simulink model "rectifire_single_inverter_pv1"  (R2022b)
settings: Solver=ode23tb  StartTime=0  StopTime=3  RelTol=1e-4
undefined symbols (not defined in the file): Ion, Lithium, P_100, sigbuilder_block, time_step
libraries: spsSeriesRLCBranchLib x26, spsTriangleGeneratorLib x26, slpidlib x26, spsVoltageMeasurementLib x14, spsCurrentMeasurementLib x11, spsDiodeLib x9, simulink x8, spsIGBTDiodeLib x8, spsMosfetLib x8, powerlib_extras x4, spsGroundLib x2, spsBatteryLib x2
(part 6 of 6)

== matlab function rectifire_single_inverter_pv1/battery/Battery and DC-DC converter/MATLAB Function7 ==
  settings: updateMethod=DISCRETE
  data: iL_ref input; u1 output; iL input; vc_ref input; vc input; vin input; i_out input; Ts input; u2 output; Bus_load input
function [u1, u2] = Passivity_BC(iL_ref, iL, vc_ref, vc, vin, i_out, Ts, Bus_load)
% Constant output voltage Module
%   param vc_ref: expected
%   param vc: dcdc output voltage
%   param vin: input voltage
%   param io: current in output side
%   param Bus_load:
%% system parameters
L = 40e-6;  % Inductance 电感 20uH
L_DMinductor = 2.2e-6;
L = L + L_DMinductor;
RL = 0.004;
Co = 1440e-6;  % 电容大小

zeta1 = L / RL * 2000;  % dumping gains
zeta2 = Co * 1000; 

% if Bus_load > 1e4
%     zeta2 = 1e-3;
% end


% error functions: state variable
x1 = iL - iL_ref;
x2 = vc - vc_ref;
persistent iL_ref_old vc_ref_old;
if isempty(iL_ref_old)
    iL_ref_old = 0;
    vc_ref_old = 0;
end

diL_ref = (iL_ref - iL_ref_old) / Ts;
dvc_ref = (vc_ref - vc_ref_old) / Ts;
%% calculate switching signal: u1,u2
% u2 denotes S3's state
% u1 denotes S1's state
u2 = 1 / iL_ref * (iL_ref - dvc_ref * Co - i_out + x2*zeta2);
u1 = 1 / vin * (L*diL_ref + RL*iL_ref + vc_ref*(1-u2) - x1*zeta1);
iL_ref_old = iL_ref;
vc_ref_old = vc_ref;

% compensate strategy
S1_duty_cycle = vc_ref / vin;
S4_duty_cycle = 1 - vin / vc_ref;  % vin < vc
S3_duty_cycle = 1- S4_duty_cycle;
PWM_triangular_wave_range = 2;
PWM_triangular_wave_min = -1;
original_u2 = u2;


persistent voltage_surge_max;
if isempty(voltage_surge_max)
    voltage_surge_max = 0;
end

if Bus_load > 1e2
    u2 = S4_duty_cycle;  % need to check
end

% if Bus_load > 1e2 && abs(vc - vc_ref) < 0.2
%     u2 = 0.5 * PWM_triangular_wave_range + PWM_triangular_wave_min;
%     u1 = 0.5 * PWM_triangular_wave_range + PWM_triangular_wave_min;
% end

if vc - vc_ref > 1 && (vc - voltage_surge_max > -0.4)
%     u2 = 2;
    u2 = S3_duty_cycle * PWM_triangular_wave_range + PWM_triangular_wave_min;
end
if vc - vc_ref > 1 && vin - vc_ref > 1
    u1 = (1 - S1_duty_cycle) * PWM_triangular_wave_range + PWM_triangular_wave_min;
end

% solve buck-boost mode: sudden u2=1, keep bucking
if vc_ref -vc > 0.2 && Bus_load > 1e2
    % In buck-boost mode, start boost when vc starts to drop > 0.3V
    u2 = S4_duty_cycle;
    u1 = max(u1, S3_duty_cycle* PWM_triangular_wave_range + PWM_triangular_wave_min);
end

% % Boost mode
% if (vc_ref - vin) > 1 && (vc_ref - vc) > 0.5
%     u1 = S1_duty_cycle * PWM_triangular_wave_range + PWM_triangular_wave_min;
% %     u2 = S4_duty_cycle * PWM_triangular_wave_range + PWM_triangular_wave_min;
% end
% 
% % Buck mode
% if vin - vc_ref > 1 && vc - vc_ref > 1
%     u2 = 2;
% %     u1 = S1_duty_cycle * PWM_triangular_wave_range + PWM_triangular_wave_min;
% end

voltage_surge_max = max(vc, voltage_surge_max);

== matlab function rectifire_single_inverter_pv1/battery/Battery and DC-DC converter1/MATLAB Function ==
  settings: updateMethod=DISCRETE
  data: iL_ref input; u1 output; iL input; vc_ref input; vc input; vin input; i_out input; Ts input; u2 output; Bus_load input; i_battery input; P_full_load input
function [u1, u2] = Passivity_BC(iL_ref, iL, vc_ref, vc, vin, i_out, Ts, Bus_load, i_battery, P_full_load)
% Constant output voltage Module
%   param vc_ref: expected
%   param vc: dcdc output voltage
%   param vin: input voltage
%   param io: current in output side
%   param Bus_load:
%   param i_battery
%   param P_full_load: full load power
%% system parameters
L = 40e-6;  % Inductance 电感 20uH
% L_DMinductor = 2.2e-6;
% L = L + L_DMinductor;
RL = 0.004;
Co = 1440e-6;  % 电容大小

zeta1 = L / RL * 2000;  % dumping gains
zeta2 = Co * 1000; 

% if Bus_load > 1e4
%     zeta2 = 1e-3;
% end


% error functions: state variable
x1 = iL - iL_ref;
x2 = vc - vc_ref;
persistent iL_ref_old vc_ref_old;
if isempty(iL_ref_old)
    iL_ref_old = 0;
    vc_ref_old = 0;
end

diL_ref = (iL_ref - iL_ref_old) / Ts;
dvc_ref = (vc_ref - vc_ref_old) / Ts;
%% calculate switching signal: u1,u2
% u2 denotes S3's state
% u1 denotes S1's state
u2 = 1 / iL_ref * (iL_ref - dvc_ref * Co - i_out + x2*zeta2);
u1 = 1 / vin * (L*diL_ref + RL*iL_ref + vc_ref*(1-u2) - x1*zeta1);
iL_ref_old = iL_ref;
vc_ref_old = vc_ref;

% compensate strategy
S1_duty_cycle = vc_ref / vin;  % buck mode == (u2==0)
S4_duty_cycle = 1 - vin / vc_ref;  % boost mode (u1==1)
PWM_triangular_wave_range = 2;
PWM_triangular_wave_min = -1;

persistent voltage_surge_max;
if isempty(voltage_surge_max)
    voltage_surge_max = 0;
end

% if Bus_load < 1e-2
%     u2 = S4_duty_cycle * PWM_triangular_wave_range + PWM_triangular_wave_min;  % ok
% end

% % Modify overshoot at initial stage
% if vc - vc_ref > 1 %&& (vc - voltage_surge_max > -0.4)
%     u2 = 2;
% %     u2 = S3_duty_cycle * PWM_triangular_wave_range + PWM_triangular_wave_min;
%     if vin - vc_ref > 1
%         u1 = (1 - S1_duty_cycle) * PWM_triangular_wave_range + PWM_triangular_wave_min;
%     end
% end
% 
% BoostMode
% if vc_ref -vc > 0.5 % && Bus_load > 1e2
%     u2 = S4_duty_cycle;
% %     u2 = S3_duty_cycle * PWM_triangular_wave_range + PWM_triangular_wave_min;
%     u1 = max(u1, S3_duty_cycle* PWM_triangular_wave_range + PWM_triangular_wave_min);
% %     u1 = 2;
% end
% 
% 
% if abs(i_out) < 5 && abs(vc - vc_ref) < 0.3
%     u2 = S4_duty_cycle;
% end




% Boost mode
if (vc_ref - vc) > 0.5 % (vc_ref - vin) > 1
    u1 = PWM_triangular_wave_min + PWM_triangular_wave_range + 1;
    u2 = S4_duty_cycle * PWM_triangular_wave_range + PWM_triangular_wave_min;
end

% Buck mode
if (vc - vc_ref) > 0.5 % (vin - vc_ref > 1) &&
    u1 = S1_duty_cycle * PWM_triangular_wave_range + PWM_triangular_wave_min;
    u2 = PWM_triangular_wave_min;
end


% prevent current surge
if (Bus_load < 1e-5) || (Bus_load > 1.05 * P_full_load) ||(i_battery < -1e-1)
    u1 = PWM_triangular_wave_min; 
    u2 = PWM_triangular_wave_range + PWM_triangular_wave_min; 
end


voltage_surge_max = max(vc, voltage_surge_max);

== matlab function rectifire_single_inverter_pv1/motor/MATLAB Function ==
  data: Vd input; V output; Vq input
function V = fcn(Vd,Vq)

V=sqrt(Vd^2+Vq^2);

== matlab function rectifire_single_inverter_pv1/motor/MATLAB Function1 ==
  data: Te input; P output; n input
function P = fcn(Te,n)

P=(Te*n)/9550;

== matlab function rectifire_single_inverter_pv1/motor/MTPA ==
  data: Is input; id output; iq output
function [id,iq] = fcn(Is)

% motor perameter
Psif=0.00569;
Lq=0.000057;
Ld=0.0000323;

%Psif=0.1827;
%Lq=12e-3;
%Ld=5.25e-3;

D=Psif/(Lq-Ld);

%calculate id and iq
%id=(Psif-sqrt(Psif^2+8*(Lq-Ld)^2*Is^2))/(4*(Lq-Ld));
%iq=sqrt(Is^2-id^2);


id=0.25*D-sqrt((0.25*D)^2+0.5*Is^2);

iq=sqrt(Is^2-id^2);

== matlab function rectifire_single_inverter_pv1/motor/power calculate/MATLAB Function ==
  data: Vd input; P output; Vq input; Id input; Iq input
function P = fcn(Vd,Vq,Id,Iq)

%瞬时无功功率理论
%P=Vd.*Id+Vq.*Iq;

P=sqrt(Vd^2+Vq^2)*sqrt(Id^2+Iq^2);

== matlab function rectifire_single_inverter_pv1/battery/Battery and DC-DC converter1/MATLAB Function2 ==
  settings: updateMethod=DISCRETE
  data: iL_ref input; u1 output; iL input; i_out_ref input; i_out input; vin input; Vc input; Ts input; u2 output
function [u1, u2] = Passivity_BC(iL_ref, iL,i_out_ref, i_out, vin, Vc, Ts)
% Constant output current Module
% param iL: inductor's current
% param iL_ref: expected value of inductor's current
% param i_out: dcdc output current 
% param i_out_ref
% param vin: input voltage
% param Vc: output voltage
%% system parameters
L = 40e-6;  % Inductance 电感 20uH
L_DMinductor = 2.2e-6;
L = L + L_DMinductor;
RL = 0.004;
C_output = 1440e-6;  % 电容大小

% zeta1 = 6 * 2;  % dumping gains
% zeta2 = 0.08 * 10;
zeta1 = L / RL * 2000;  % dumping gains
zeta2 = C_output * 1000; 

% error functions: state variable
x1 = iL - iL_ref;
x2 = i_out - i_out_ref;
persistent iL_ref_old Vc_old;
if isempty(iL_ref_old)
    iL_ref_old = 0;
    Vc_old = 0;
end

diL_ref = (iL_ref - iL_ref_old) / Ts;
dVc_ref = (Vc - Vc_old) / Ts;
%% calculate switching signal: u1,u2
u2 = 1 / iL_ref * (iL_ref - C_output * dVc_ref - i_out_ref + x2*zeta2);
u1 = 1 / vin * (L*diL_ref + RL * iL_ref + Vc * (1 - u2) - x1*zeta1);

iL_ref_old = iL_ref;
Vc_old = Vc;

== matlab function rectifire_single_inverter_pv1/battery/Battery and DC-DC converter1/MATLAB Function3 ==
  settings: updateMethod=DISCRETE
  data: iL_ref input; u1 output; iL input; vc_ref input; vc input; vin input; i_out input; Ts input; u2 output
function [u1, u2] = Passivity_BC(iL_ref, iL, vc_ref, vc, vin, i_out, Ts)
% Constant output voltage Module
%   param vc_ref: expected
%   param vc: dcdc output voltage
%   param vin: input voltage
%   param io: current in output side
%% system parameters
L = 40e-6;  % Inductance 电感 20uH
L_DMinductor = 2.2e-6;
L = L + L_DMinductor;
RL = 0.004;
Co = 1440e-6;  % 电容大小

zeta1 = 6 * 2;  % dumping gains
zeta2 = 0.08 * 10; 

% error functions: state variable
x1 = iL - iL_ref;
x2 = vc - vc_ref;
persistent iL_ref_old vc_ref_old;
if isempty(iL_ref_old)
    iL_ref_old = 0;
    vc_ref_old = 0;
end

diL_ref = (iL_ref - iL_ref_old) / Ts;
dvc_ref = (vc_ref - vc_ref_old) / Ts;
%% calculate switching signal: u1,u2
u2 = 1 / iL_ref * (iL_ref - dvc_ref * Co - i_out + x2*zeta2);
u1 = 1 / vin * (L*diL_ref + RL*iL_ref + vc_ref*(1-u2) - x1*zeta1);
iL_ref_old = iL_ref;
vc_ref_old = vc_ref;

== matlab function rectifire_single_inverter_pv1/battery/Battery and DC-DC converter1/Discharge Const Voltage/MATLAB Function1 ==
  settings: updateMethod=DISCRETE
  data: iL_ref input; u1 output; iL input; vc_ref input; vc input; vin input; i_out input; Ts input; u2 output; Bus_load input; i_battery input; P_full_load input
function [u1, u2] = Passivity_BC(iL_ref, iL, vc_ref, vc, vin, i_out, Ts, Bus_load, i_battery, P_full_load)
% Constant output voltage Module
%   param vc_ref: expected
%   param vc: dcdc output voltage
%   param vin: input voltage
%   param io: current in output side
%   param Bus_load:
%   param i_battery
%   param P_full_load: full load power
%% system parameters
L = 40e-6;  % Inductance 电感 20uH
% L_DMinductor = 2.2e-6;
% L = L + L_DMinductor;
RL = 0.004;
Co = 1440e-6;  % 电容大小

zeta1 = L / RL * 2000;  % dumping gains
zeta2 = Co * 1000; 

% if Bus_load > 1e4
%     zeta2 = 1e-3;
% end


% error functions: state variable
x1 = iL - iL_ref;
x2 = vc - vc_ref;
persistent iL_ref_old vc_ref_old;
if isempty(iL_ref_old)
    iL_ref_old = 0;
    vc_ref_old = 0;
end

diL_ref = (iL_ref - iL_ref_old) / Ts;
dvc_ref = (vc_ref - vc_ref_old) / Ts;
%% calculate switching signal: u1,u2
% u2 denotes S3's state
% u1 denotes S1's state
u2 = 1 / iL_ref * (iL_ref - dvc_ref * Co - i_out + x2*zeta2);
u1 = 1 / vin * (L*diL_ref + RL*iL_ref + vc_ref*(1-u2) - x1*zeta1);
iL_ref_old = iL_ref;
vc_ref_old = vc_ref;

% compensate strategy
S1_duty_cycle = vc_ref / vin;  % buck mode == (u2==0)
S4_duty_cycle = 1 - vin / vc_ref;  % boost mode (u1==1)
S3_duty_cycle = 1- S4_duty_cycle;
PWM_triangular_wave_range = 2;
PWM_triangular_wave_min = -1;
original_u2 = u2;


persistent voltage_surge_max;
if isempty(voltage_surge_max)
    voltage_surge_max = 0;
end

if Bus_load > 1e2
    u2 = S4_duty_cycle * PWM_triangular_wave_range + PWM_triangular_wave_min;;  % ok
end

% % Modify overshoot at initial stage
% if vc - vc_ref > 1 %&& (vc - voltage_surge_max > -0.4)
%     u2 = 2;
% %     u2 = S3_duty_cycle * PWM_triangular_wave_range + PWM_triangular_wave_min;
%     if vin - vc_ref > 1
%         u1 = (1 - S1_duty_cycle) * PWM_triangular_wave_range + PWM_triangular_wave_min;
%     end
% end
% 
% % % BoostMode
% % if vc_ref -vc > 0.5 % && Bus_load > 1e2
% %     u2 = S4_duty_cycle;
% % %     u2 = S3_duty_cycle * PWM_triangular_wave_range + PWM_triangular_wave_min;
% %     u1 = max(u1, S3_duty_cycle* PWM_triangular_wave_range + PWM_triangular_wave_min);
% % %     u1 = 2;
% % end
% 
% 
% if abs(i_out) < 5 && abs(vc - vc_ref) < 0.3
%     u2 = S4_duty_cycle;
% end




% Boost mode
if (vc_ref - vc) > 0.5 % (vc_ref - vin) > 1
    u1 = PWM_triangular_wave_min + PWM_triangular_wave_range;
    u2 = S4_duty_cycle * PWM_triangular_wave_range + PWM_triangular_wave_min;
end

% Buck mode
if (vc - vc_ref) > 0.5 % (vin - vc_ref > 1) &&
    u1 = S1_duty_cycle * PWM_triangular_wave_range + PWM_triangular_wave_min;
    u2 = PWM_triangular_wave_min;
end

% prevent current surge
if (Bus_load < 1e-5) || (Bus_load > 1.05 * P_full_load) ||(i_battery < 1e-10) ...
        || (i_out < 1e-10) || (vc > vc_ref + 20)
    % (vc > vc_ref + 20) the voltage is too big, could not operate buck
    % normally and may cause current inverse
    u1 = PWM_triangular_wave_min; 
    u2 = PWM_triangular_wave_range + PWM_triangular_wave_min; 
end

voltage_surge_max = max(vc, voltage_surge_max);

== matlab function rectifire_single_inverter_pv1/battery/Battery and DC-DC converter1/MATLAB Function5 ==
  settings: updateMethod=DISCRETE
  data: iL_ref input; u1 output; iL input; i_out_ref input; i_out input; vin input; Vc input; Ts input; u2 output
function [u1, u2] = Passivity_BC(iL_ref, iL,i_out_ref, i_out, vin, Vc, Ts)
% Constant output current Module
% param iL: inductor's current
% param iL_ref: expected value of inductor's current
% param i_out: dcdc output current 
% param i_out_ref
% param vin: input voltage
% param Vc: output voltage
%% system parameters
L = 40e-6;  % Inductance 电感 20uH
L_DMinductor = 2.2e-6;
L = L + L_DMinductor;
RL = 0.004;
C_output = 1440e-6;  % 电容大小

zeta1 = 6;  % dumping gains
zeta2 = 0.08;

% error functions: state variable
x1 = iL - iL_ref;
x2 = i_out - i_out_ref;
persistent iL_ref_old Vc_old;
if isempty(iL_ref_old)
    iL_ref_old = 0;
    Vc_old = 0;
end

diL_ref = (iL_ref - iL_ref_old) / Ts;
dVc_ref = (Vc - Vc_old) / Ts;
%% calculate switching signal: u1,u2
u2 = 1 / iL_ref * (iL_ref - C_output * dVc_ref - i_out_ref + x2*zeta2);
u1 = 1 / vin * (L*diL_ref + RL * iL_ref + Vc * (1 - u2) - x1*zeta1);

iL_ref_old = iL_ref;
Vc_old = Vc;
